simulink model "sampleModel1488"  (R2023a)
settings: Solver=VariableStepAuto  StartTime=0.0  StopTime=10.0  RelTol=1e-3
libraries: simulink x5, hdlsllib x5
settings Model: Creator=user1  LastModifiedBy=user1

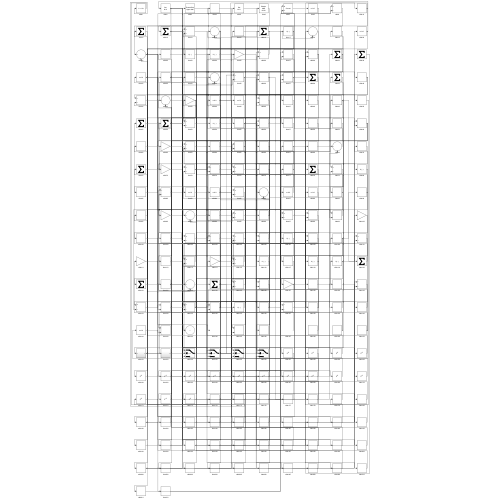
[thumbnail: Simulink's stored preview of the top-level diagram]
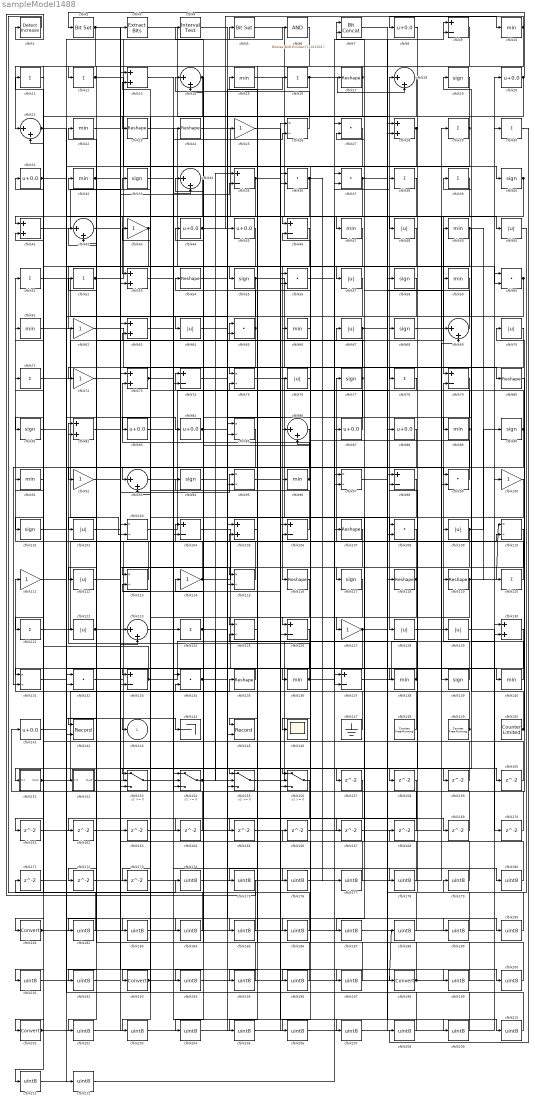
== system sampleModel1488 ==
  cfblk1 : simulink/Logic and Bit Operations/Detect Increase  vinit=0.0  OutDataTypeStr=boolean
      settings: LibrarySourceBlock=|
      | hdlsllib/Logic and Bit
      | Operations/Detect
      | Increase
  cfblk{10,15,22,32,47,49,59,61,66,89,91,96,136,138,140} (15 alike) : MinMax
  cfblk{25,43,62,72,92,100,111,114,127} (9 alike) : Gain
  cfblk{19,33,40,55,58,68,77,81,90,94,101,117,139} (13 alike) : Signum
  cfblk{48,50,57,64,67,70,76,102,109,112,122,128..129} (13 alike) : Abs  SaturateOnIntegerOverflow=off
  cfblk{26,75,85,95,97,103,110,113,115,125,131} (11 alike) : Product  Inputs=*/  RndMeth=Zero  SaturateOnIntegerOverflow=on
  cfblk{9,35,46,74,79,98,104,106,126,133,137} (11 alike) : Sum  Inputs=+-
  cfblk{13,28,41,53,63,73,82,105,130} (9 alike) : Sum
  cfblk{17,23..24,54,80,107,116,118..119,135} (10 alike) : Reshape
  cfblk{27,36..37,56,60,65,99,108,132,134} (10 alike) : DotProduct  OutDataTypeStr=Inherit: Inherit via internal rule
  cfblk{11..12,16,29..30,38..39,51..52,71,78,120..121,124} (14 alike) : Sum  Inputs=+
  cfblk{14,18,21,34,42,69,86,93,123} (9 alike) : Sum  Inputs=|++
  cfblk{8,20,31,44..45,83..84,87..88,141} (10 alike) : Bias  Bias=0.0  SaturateOnIntegerOverflow=off
  cfblk142 : Record  FileSettingsInternal="{\"entries\":[{\"content\":{\"excelSettings\":{\"content\":{},\"type\":\"Streamout.ExcelSettings\"}},\"type\":\"Streamout.FileSettingStorage\",\"uuid\":\"\"}],\"packageUris\":[\"http:\\/\\/schema.mathworks.com\\/mf0\\/streamout_blocks\\/R2020a\"],\"version\":\"1.0\"}"  Layout=[1 1]  SignalsInternal="{\"entries\":[{\"content\":{\"signals\":[{\"content\":{\"blockPath\":[],\"dimensions\":[1],\"domain\":\"\",\"lineColor\":\"#a2142f\",\"plots\":[1],\"port\":1,\"signalID\":1193,\"signalName\":\"XY Graph:1\"},\"type\":\"RecordBlkView.Signal\",\"uuid\":\"\"},{\"content\":{\"blockPath\":[],\"dimensions\":[1],\"domain\":\"\",\"lineColor\":\"#139fff\",\"plots\":[1],\"port\":2,\"signalID\":1196,\"signalName\":\"XY Graph:2\"},\"type\":\"RecordBlkView.Signal\",\"uuid\":\"\"}]},\"type\":\"RecordBlkView.InputSignals\",\"uuid\":\"\"}],\"packageUris\":[\"http:\\/\\/schema.mathworks.com\\/mf0\\/streamout_blocks\\/R2020a\"],\"version\":\"1.0\"}"  VisualizationBindings="{\"xyplotplugin\":{\"info\":[{\"series\":[{\"bindingParametersList\":[{\"parameter\":\"X-Axis\",\"signalID\":1193,\"signalName\":\"XY Graph:1\"},{\"parameter\":\"Y-Axis\",\"signalID\":1196,\"signalName\":\"XY Graph:2\"}],\"seriesID\":30784}],\"subplotID\":1}]}}"  CompatibilityTag=XY  st=-1
  cfblk144 : Terminator
  cfblk145 : Record  FileSettingsInternal="{\"entries\":[{\"content\":{\"excelSettings\":{\"content\":{},\"type\":\"Streamout.ExcelSettings\"}},\"type\":\"Streamout.FileSettingStorage\",\"uuid\":\"\"}],\"packageUris\":[\"http:\\/\\/schema.mathworks.com\\/mf0\\/streamout_blocks\\/R2020a\"],\"version\":\"1.0\"}"  Layout=[1 1]  SignalsInternal="{\"entries\":[{\"content\":{\"signals\":[{\"content\":{\"blockPath\":[],\"dimensions\":[1],\"domain\":\"\",\"lineColor\":\"#a2142f\",\"plots\":[1],\"port\":1,\"signalID\":1201,\"signalName\":\"XY Graph:1\"},\"type\":\"RecordBlkView.Signal\",\"uuid\":\"\"},{\"content\":{\"blockPath\":[],\"dimensions\":[1],\"domain\":\"\",\"lineColor\":\"#139fff\",\"plots\":[1],\"port\":2,\"signalID\":1204,\"signalName\":\"XY Graph:2\"},\"type\":\"RecordBlkView.Signal\",\"uuid\":\"\"}]},\"type\":\"RecordBlkView.InputSignals\",\"uuid\":\"\"}],\"packageUris\":[\"http:\\/\\/schema.mathworks.com\\/mf0\\/streamout_blocks\\/R2020a\"],\"version\":\"1.0\"}"  VisualizationBindings="{\"xyplotplugin\":{\"info\":[{\"series\":[{\"bindingParametersList\":[{\"parameter\":\"X-Axis\",\"signalID\":1201,\"signalName\":\"XY Graph:1\"},{\"parameter\":\"Y-Axis\",\"signalID\":1204,\"signalName\":\"XY Graph:2\"}],\"seriesID\":31207}],\"subplotID\":1}]}}"  CompatibilityTag=XY  st=-1
  cfblk146 : Scope
  cfblk147 : Ground
  cfblk148 : hdlsllib/Sources/Counter Free-Running  NumBits=16  tsamp=-1
  cfblk149 : hdlsllib/Sources/Counter Free-Running  NumBits=16  tsamp=-1
  cfblk150 : hdlsllib/Sources/Counter Limited  uplimit=7  tsamp=-1
  cfblk151 : Subsystem
      settings: LibrarySourceBlock=|
      | hdlsllib/Ports &
      | Subsystems/Subsystem
  cfblk152 : Subsystem
      settings: LibrarySourceBlock=|
      | hdlsllib/Ports &
      | Subsystems/Subsystem
  cfblk{153..156} (4 alike) : Switch  SaturateOnIntegerOverflow=off  InputSameDT=off
  cfblk{157..173} (17 alike) : Delay  SampleTime=1
  cfblk{174..180,182..192,194..197,199..200,202..212} (35 alike) : DataTypeConversion  OutDataTypeStr=uint8  SaturateOnIntegerOverflow=off  RndMeth=Floor
  cfblk{181,193,198,201} (4 alike) : DataTypeConversion  SaturateOnIntegerOverflow=off  RndMeth=Floor
  cfblk2 : simulink/Logic and Bit Operations/Bit Set  iBit=0
      settings: LibrarySourceBlock=|
      | hdlsllib/Logic and Bit
      | Operations/Bit Set
  cfblk3 : simulink/Logic and Bit Operations/Extract Bits  bitsToExtract=Upper half  numBits=8  bitIdxRange=[0 7]  outScalingMode=Preserve fixed-point scaling
      settings: LibrarySourceBlock=|
      | hdlsllib/Logic and Bit
      | Operations/Extract Bits
  cfblk4 : hdlsllib/Logic and Bit Operations/Interval Test  IntervalClosedRight=on  uplimit=0.5  IntervalClosedLeft=on  lowlimit=-0.5  OutDataTypeStr=boolean
  cfblk5 : simulink/Logic and Bit Operations/Bit Set  iBit=0
      settings: LibrarySourceBlock=|
      | hdlsllib/Logic and Bit
      | Operations/Bit Set
  cfblk6 : simulink/Logic and Bit Operations/Bitwise Operator  logicop=AND  UseBitMask=on  BitMask=bin2dec('11011001')  BitMaskRealWorld=Stored Integer
      settings: LibrarySourceBlock=|
      | hdlsllib/Logic and Bit
      | Operations/Bitwise
      | Operator
  cfblk7 : hdlsllib/Logic and Bit Operations/Bit Concat  numInputs=2
  cfblk143 : Outport  VectorParamsAs1DForOutWhenUnconnected=off
  wires:
  cfblk85/1 -> cfblk201/1
  cfblk122/1 -> cfblk18/1, cfblk35/2
  cfblk61/1 -> cfblk103/2
  cfblk117/1 -> cfblk82/1
  cfblk99/1 -> cfblk54/1
  cfblk53/1 -> cfblk57/1
  cfblk2/1 -> cfblk21/1, cfblk154/3, cfblk56/2, cfblk65/2
  cfblk147/1 -> cfblk111/1
  cfblk124/1 -> cfblk155/2, cfblk157/1
  cfblk44/1 -> cfblk10/1, cfblk189/1
  cfblk47/1 -> cfblk55/1
  cfblk60/1 -> cfblk151/1(In1), cfblk83/1, cfblk142/2
  cfblk39/1 -> cfblk79/1
  cfblk135/1 -> cfblk131/1
  cfblk56/1 -> cfblk38/1
  cfblk120/1 -> cfblk77/1
  cfblk90/1 -> cfblk74/1, cfblk115/1
  cfblk36/1 -> cfblk46/1, cfblk177/1
  cfblk20/1 -> cfblk2/1, cfblk145/1
  cfblk46/1 -> cfblk62/1
  cfblk23/1 -> cfblk116/1
  cfblk15/1 -> cfblk139/1
  cfblk114/1 -> cfblk82/2, cfblk88/1
  cfblk103/1 -> cfblk68/1
  cfblk104/1 -> cfblk140/1
  cfblk55/1 -> cfblk78/1, cfblk142/1, cfblk209/1
  cfblk115/1 -> cfblk51/1
  cfblk25/1 -> cfblk106/1
  cfblk151/1(Out1) -> cfblk135/1, cfblk184/1
  cfblk128/1 -> cfblk79/2
  cfblk80/1 -> cfblk141/1
  cfblk75/1 -> cfblk128/1
  cfblk106/1 -> cfblk32/1
  cfblk42/1 -> cfblk198/1
  cfblk140/1 -> cfblk39/1
  cfblk139/1 -> cfblk119/1
  cfblk93/1 -> cfblk96/1
  cfblk154/1 -> cfblk45/1, cfblk35/1, cfblk167/1
  cfblk16/1 -> cfblk18/2, cfblk121/1
  cfblk132/1 -> cfblk24/1
  cfblk6/1 -> cfblk101/1
  cfblk102/1 -> cfblk95/1
  cfblk62/1 -> cfblk107/1
  cfblk121/1 -> cfblk109/1
  cfblk12/1 -> cfblk40/1, cfblk138/1
  cfblk37/1 -> cfblk66/1, cfblk9/2
  cfblk52/1 -> cfblk5/1, cfblk115/2
  cfblk43/1 -> cfblk153/3, cfblk211/1
  cfblk5/1 -> cfblk137/1
  cfblk89/1 -> cfblk44/1, cfblk131/2
  cfblk3/1 -> cfblk58/1
  cfblk71/1 -> cfblk29/1
  cfblk48/1 -> cfblk75/1
  cfblk18/1 -> cfblk93/1
  cfblk28/1 -> cfblk113/1, cfblk146/1
  cfblk45/1 -> cfblk112/1
  cfblk150/1 -> cfblk19/1, cfblk70/1
  cfblk14/1 -> cfblk104/2, cfblk194/1
  cfblk152/1(Out1) -> cfblk26/1
  cfblk108/1 -> cfblk106/2
  cfblk78/1 -> cfblk75/2
  cfblk107/1 -> cfblk153/1
  cfblk86/1 -> cfblk95/2
  cfblk51/1 -> cfblk74/2
  cfblk17/1 -> cfblk12/1, cfblk41/1, cfblk64/1
  cfblk33/1 -> cfblk124/1
  cfblk110/1 -> cfblk117/1
  cfblk49/1 -> cfblk89/1, cfblk120/1, cfblk172/1
  cfblk40/1 -> cfblk93/2, cfblk173/1
  cfblk87/1 -> cfblk33/1
  cfblk58/1 -> cfblk76/1
  cfblk38/1 -> cfblk53/1
  cfblk27/1 -> cfblk53/2
  cfblk21/1 -> cfblk143/1, cfblk99/1, cfblk99/2
  cfblk101/1 -> cfblk152/1(In1)
  cfblk41/1 -> cfblk3/1
  cfblk88/1 -> cfblk126/1
  cfblk54/1 -> cfblk86/1
  cfblk113/1 -> cfblk71/1
  cfblk155/1 -> cfblk17/1
  cfblk35/1 -> cfblk169/1, cfblk191/1
  cfblk148/1 -> cfblk91/1
  cfblk136/1 -> cfblk122/1, cfblk9/1
  cfblk91/1 -> cfblk61/1
  cfblk149/1 -> cfblk43/1, cfblk114/1
  cfblk96/1 -> cfblk73/2, cfblk14/2
  cfblk68/1 -> cfblk49/1
  cfblk26/1 -> cfblk14/1
  cfblk24/1 -> cfblk47/1
  cfblk109/1 -> cfblk155/1, cfblk90/1, cfblk127/1
  cfblk31/1 -> cfblk48/1, cfblk60/2
  cfblk84/1 -> cfblk108/1, cfblk16/1
  cfblk119/1 -> cfblk110/1, cfblk145/2
  cfblk133/1 -> cfblk28/1, cfblk34/2, cfblk41/2
  cfblk32/1 -> cfblk50/1, cfblk156/2
  cfblk127/1 -> cfblk59/1, cfblk192/1
  cfblk73/1 -> cfblk69/1, cfblk80/1
  cfblk10/1 -> cfblk8/1, cfblk182/1
  cfblk19/1 -> cfblk81/1
  cfblk57/1 -> cfblk92/1
  cfblk138/1 -> cfblk27/2, cfblk125/2
  cfblk81/1 -> cfblk84/1
  cfblk72/1 -> cfblk144/1
  cfblk70/1 -> cfblk86/2
  cfblk126/1 -> cfblk133/1
  cfblk118/1 -> cfblk126/2, cfblk15/1
  cfblk69/1 -> cfblk7/1
  cfblk137/1 -> cfblk30/1
  cfblk67/1 -> cfblk125/1, cfblk160/1
  cfblk125/1 -> cfblk65/1
  cfblk100/1 -> cfblk193/1
  cfblk65/1 -> cfblk102/1, cfblk34/1
  cfblk77/1 -> cfblk52/1, cfblk137/2
  cfblk153/1 -> cfblk26/2
  cfblk29/1 -> cfblk23/1, cfblk132/2, cfblk72/1
  cfblk94/1 -> cfblk25/1
  cfblk7/1 -> cfblk118/1
  cfblk92/1 -> cfblk154/2
  cfblk83/1 -> cfblk156/1
  cfblk111/1 -> cfblk136/1
  cfblk134/1 -> cfblk94/1, cfblk110/2, cfblk104/1
  cfblk11/1 -> cfblk181/1
  cfblk131/1 -> cfblk6/1
  cfblk8/1 -> cfblk158/1
  cfblk95/1 -> cfblk159/1
  cfblk159/1 -> cfblk21/2
  cfblk160/1 -> cfblk134/1
  cfblk34/1 -> cfblk161/1
  cfblk161/1 -> cfblk133/2
  cfblk156/1 -> cfblk162/1
  cfblk162/1 -> cfblk69/2
  cfblk82/1 -> cfblk163/1
  cfblk163/1 -> cfblk37/2
  cfblk79/1 -> cfblk164/1
  cfblk164/1 -> cfblk73/1
  cfblk9/1 -> cfblk165/1
  cfblk166/1 -> cfblk46/2
  cfblk167/1 -> cfblk7/2
  cfblk168/1 -> cfblk154/1
  cfblk169/1 -> cfblk113/2
  cfblk129/1 -> cfblk170/1
  cfblk170/1 -> cfblk36/1
  cfblk172/1 -> cfblk28/2
  cfblk173/1 -> cfblk155/3
  cfblk1/1 -> cfblk174/1
  cfblk174/1 -> cfblk87/1
  cfblk157/1 -> cfblk175/1
  cfblk175/1 -> cfblk1/1
  cfblk4/1 -> cfblk176/1
  cfblk176/1 -> cfblk129/1
  cfblk177/1 -> cfblk4/1
  cfblk13/1 -> cfblk178/1
  cfblk178/1 -> cfblk67/1
  cfblk50/1 -> cfblk179/1
  cfblk179/1 -> cfblk13/1
  cfblk64/1 -> cfblk180/1
  cfblk180/1 -> cfblk13/2
  cfblk181/1 -> cfblk36/2, cfblk197/1
  cfblk182/1 -> cfblk11/1
  cfblk171/1 -> cfblk183/1
  cfblk183/1 -> cfblk60/1
  cfblk184/1 -> cfblk171/1
  cfblk22/1 -> cfblk185/1
  cfblk185/1 -> cfblk31/1
  cfblk74/1 -> cfblk186/1
  cfblk186/1 -> cfblk22/1
  cfblk98/1 -> cfblk187/1
  cfblk187/1 -> cfblk20/1
  cfblk188/1 -> cfblk98/1
  cfblk189/1 -> cfblk98/2
  cfblk123/1 -> cfblk190/1
  cfblk190/1 -> cfblk168/1
  cfblk191/1 -> cfblk123/1
  cfblk192/1 -> cfblk123/2
  cfblk193/1 -> cfblk188/1, cfblk156/3
  cfblk194/1 -> cfblk100/1
  cfblk105/1 -> cfblk195/1
  cfblk195/1 -> cfblk134/2
  cfblk66/1 -> cfblk196/1
  cfblk196/1 -> cfblk105/1
  cfblk197/1 -> cfblk105/2
  cfblk198/1 -> cfblk166/1, cfblk37/1
  cfblk165/1 -> cfblk199/1
  cfblk199/1 -> cfblk42/1
  cfblk112/1 -> cfblk200/1
  cfblk200/1 -> cfblk42/2
  cfblk201/1 -> cfblk153/2, cfblk56/1, cfblk103/1
  cfblk158/1 -> cfblk202/1
  cfblk202/1 -> cfblk85/1
  cfblk116/1 -> cfblk203/1
  cfblk203/1 -> cfblk85/2
  cfblk130/1 -> cfblk204/1
  cfblk204/1 -> cfblk27/1
  cfblk59/1 -> cfblk205/1
  cfblk205/1 -> cfblk130/1
  cfblk76/1 -> cfblk206/1
  cfblk206/1 -> cfblk130/2
  cfblk63/1 -> cfblk207/1
  cfblk207/1 -> cfblk108/2
  cfblk30/1 -> cfblk208/1
  cfblk208/1 -> cfblk63/1
  cfblk209/1 -> cfblk63/2
  cfblk97/1 -> cfblk210/1
  cfblk210/1 -> cfblk132/1
  cfblk211/1 -> cfblk97/1
  cfblk141/1 -> cfblk212/1
  cfblk212/1 -> cfblk97/2

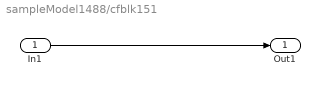
== system sampleModel1488/cfblk151 ==
  In1 : Inport
  Out1 : Outport
  wires:
  In1/1 -> Out1/1

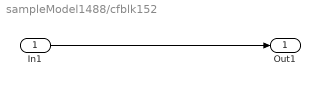
== system sampleModel1488/cfblk152 ==
  In1 : Inport
  Out1 : Outport
  wires:
  In1/1 -> Out1/1
